simulink library "SIXOSEM_F_STAGE_MONITOR_MASTER"  (Simulink 8.0)
settings: Solver=ode45  StartTime=0.0  StopTime=10.0  RelTol=1e-3
libraries: SIXOSEM_F_MONITOR_MASTER x4
settings Model: Creator=controls  LastModifiedBy=controls

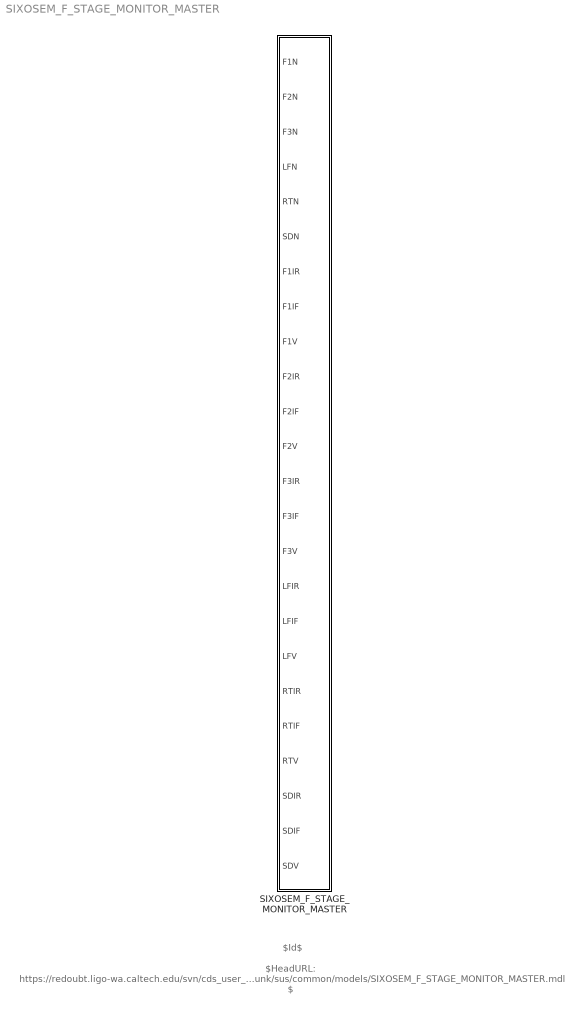
== system SIXOSEM_F_STAGE_MONITOR_MASTER ==
  note: $HeadURL: https://redoubt.ligo-wa.caltech.edu/svn/cds_user_apps/trunk/sus/common/models/SIXOSEM_F_STAGE_MONITOR_MASTER.mdl $
  note: $Id$
  SIXOSEM_F_STAGE_MONITOR_MASTER : Subsystem

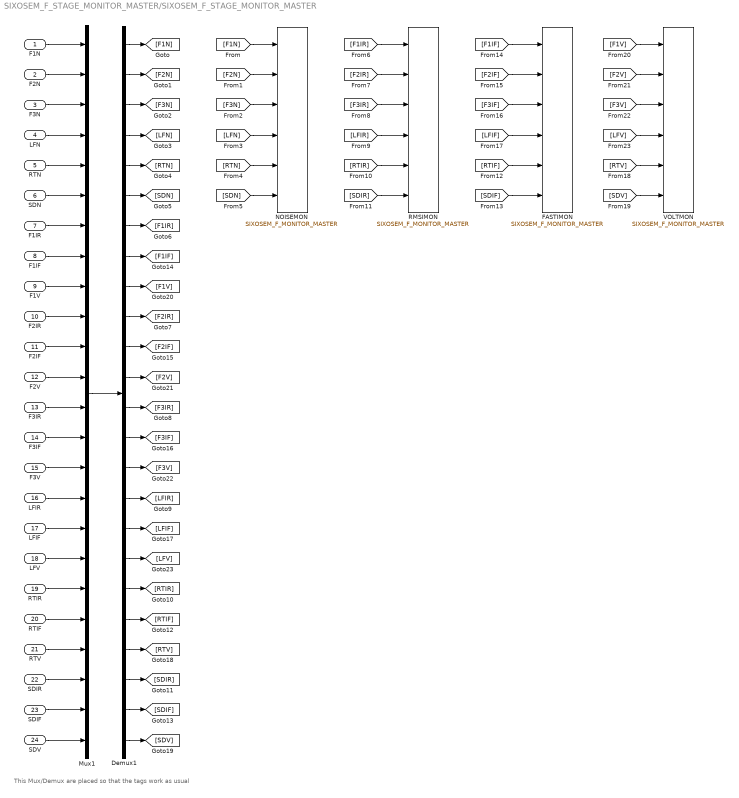
== system SIXOSEM_F_STAGE_MONITOR_MASTER/SIXOSEM_F_STAGE_MONITOR_MASTER ==
  note: This Mux/Demux are placed
      | so that the tags work as usual
  F1N : Inport
  F2N : Inport  Port=2
  F3N : Inport  Port=3
  LFN : Inport  Port=4
  RTN : Inport  Port=5
  SDN : Inport  Port=6
  F1IR : Inport  Port=7
  F1IF : Inport  Port=8
  F1V : Inport  Port=9
  F2IR : Inport  Port=10
  F2IF : Inport  Port=11
  F2V : Inport  Port=12
  F3IR : Inport  Port=13
  F3IF : Inport  Port=14
  F3V : Inport  Port=15
  LFIR : Inport  Port=16
  LFIF : Inport  Port=17
  LFV : Inport  Port=18
  RTIR : Inport  Port=19
  RTIF : Inport  Port=20
  RTV : Inport  Port=21
  SDIR : Inport  Port=22
  SDIF : Inport  Port=23
  SDV : Inport  Port=24
  Demux1 : Demux  Outputs=24
  FASTIMON : SIXOSEM_F_MONITOR_MASTER/SIXOSEM_F_MONITOR_MASTER
  Mux1 : Mux  Inputs=24
  NOISEMON : SIXOSEM_F_MONITOR_MASTER/SIXOSEM_F_MONITOR_MASTER
  RMSIMON : SIXOSEM_F_MONITOR_MASTER/SIXOSEM_F_MONITOR_MASTER
  VOLTMON : SIXOSEM_F_MONITOR_MASTER/SIXOSEM_F_MONITOR_MASTER
  wires:
  F1N/1 -> Mux1/1
  SDV/1 -> Mux1/24
  SDIF/1 -> Mux1/23
  SDIR/1 -> Mux1/22
  F2V/1 -> Mux1/12
  F3IR/1 -> Mux1/13
  F3IF/1 -> Mux1/14
  F3V/1 -> Mux1/15
  LFIR/1 -> Mux1/16
  LFIF/1 -> Mux1/17
  LFV/1 -> Mux1/18
  RTIR/1 -> Mux1/19
  RTIF/1 -> Mux1/20
  RTV/1 -> Mux1/21
  F2N/1 -> Mux1/2
  F3N/1 -> Mux1/3
  LFN/1 -> Mux1/4
  RTN/1 -> Mux1/5
  SDN/1 -> Mux1/6
  F1IR/1 -> Mux1/7
  F1IF/1 -> Mux1/8
  F1V/1 -> Mux1/9
  F2IR/1 -> Mux1/10
  F2IF/1 -> Mux1/11
  Mux1/1 -> Demux1/1
  [F1N] -> NOISEMON/1
  Demux1/1 -> [F1N]
  Demux1/2 -> [F2N]
  Demux1/3 -> [F3N]
  Demux1/4 -> [LFN]
  Demux1/5 -> [RTN]
  Demux1/6 -> [SDN]
  [F2N] -> NOISEMON/2
  [F3N] -> NOISEMON/3
  [RTN] -> NOISEMON/5
  [SDN] -> NOISEMON/6
  [LFN] -> NOISEMON/4
  [F1IR] -> RMSIMON/1
  [F2IR] -> RMSIMON/2
  [F3IR] -> RMSIMON/3
  [RTIR] -> RMSIMON/5
  [SDIR] -> RMSIMON/6
  [LFIR] -> RMSIMON/4
  Demux1/7 -> [F1IR]
  Demux1/8 -> [F1IF]
  Demux1/9 -> [F1V]
  Demux1/10 -> [F2IR]
  Demux1/11 -> [F2IF]
  Demux1/12 -> [F2V]
  Demux1/13 -> [F3IR]
  Demux1/14 -> [F3IF]
  Demux1/15 -> [F3V]
  Demux1/16 -> [LFIR]
  Demux1/17 -> [LFIF]
  Demux1/18 -> [LFV]
  Demux1/19 -> [RTIR]
  Demux1/20 -> [RTIF]
  Demux1/21 -> [RTV]
  Demux1/22 -> [SDIR]
  Demux1/23 -> [SDIF]
  Demux1/24 -> [SDV]
  [F1IF] -> FASTIMON/1
  [F2IF] -> FASTIMON/2
  [F3IF] -> FASTIMON/3
  [RTIF] -> FASTIMON/5
  [SDIF] -> FASTIMON/6
  [LFIF] -> FASTIMON/4
  [F1V] -> VOLTMON/1
  [F2V] -> VOLTMON/2
  [F3V] -> VOLTMON/3
  [RTV] -> VOLTMON/5
  [SDV] -> VOLTMON/6
  [LFV] -> VOLTMON/4
